simulink model "ch7example10"  (Simulink 5.0)
settings: Solver=FixedStepDiscrete  StartTime=0.0  StopTime=50  FixedStep=1e-4  RelTol=1e-3
undefined symbols (not defined in the file): rcosine
libraries: dspsigops x4, commsink2 x2, dspswit3 x1, dsparch4 x1, commcontsrc2 x1, simulink x1, commrandsrc2 x1, commutil2 x1
settings Model: LastModifiedBy=shaoyubin

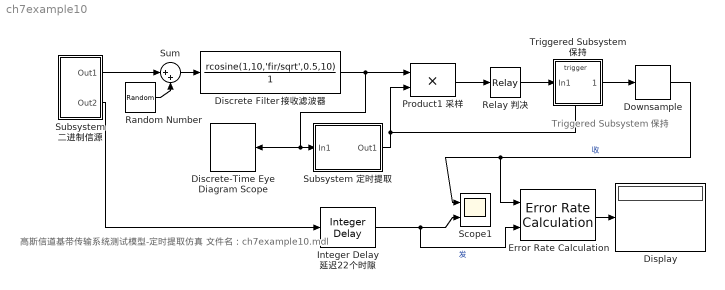
== system ch7example10 ==
  note: 高斯信道基带传输系统测试模型-定时提取仿真
      | 文件名：ch7example10.mdl
  note: Triggered
      | Subsystem
      | 保持
  Discrete Filter 接收滤波器 : DiscreteFilter  Numerator=rcosine(1,10,'fir/sqrt',0.5,10)  Denominator=1  SampleTime=1/10000
  Discrete-Time Eye Diagram Scope : commsink2/Discrete-Time Eye Diagram Scope  Tag=EyeDiagram  Orientation=left  showPlotting=on  sampPerSymb=10  offsetEye=0  symbPerTrace=2  numTraces=80  numNewFrames=80  showRendering=off  LineStyles=-  LineColors=b  dupPoints=on  fading=off  render=on  AxisGrid=on  showAxes=off  yMin=-2.17080016151619  yMax=2.13569726270215  inphaseLabel=In-phase Amplitude  quadratureLabel=Quadrature Amplitude  showFigure=off  openScopeAtSimStart=on  dispDiagram=In-phase Only  FrameNumber=on  FigPos=[76 76 560 487]  figTitle=Eye Diagram  block_type_=eye  numLinesMax=8
  Display : Display
  Downsample : dspsigops/Downsample  N=10  phase=0  ic=0  smode=Allow multirate  fmode=Maintain input frame size
  Error Rate Calculation : commsink2/Error Rate Calculation  N=0  st_delay=1  cp_mode=Entire frame  subframe=[]  PMode=Port  WsName=ErrorVec  RsMode2=off  stop=off  numErr=100  maxBits=1e6
  Integer Delay 延迟22个时隙 : dspsigops/Integer Delay  delay=22  ic=0  reset_popup=None
  Product1 采样 : Product  SaturateOnIntegerOverflow=on
  Random Number : RandomNumber  Variance=0.01  SampleTime=0
  Relay 判决 : Relay  OnSwitchValue=0  OffSwitchValue=0
  Scope1 : Scope  NumInputPorts=2
      settings: TimeRange=0.04  YMin=-2~-2  YMax=2~2
  Subsystem 定时提取 : Subsystem
  Subsystem 二进制信源 : Subsystem
  Sum : Sum  Inputs=|++  SaturateOnIntegerOverflow=on
  Triggered Subsystem 保持 : Subsystem  TreatAsAtomicUnit=on
  wires:
  Product1 采样/1 -> Relay 判决/1
  Triggered Subsystem 保持/1(Out1) -> Downsample/1
  Relay 判决/1 -> Triggered Subsystem 保持/1(In1)
  Integer Delay 延迟22个时隙/1 -> Scope1/2, Error Rate Calculation/2  "发"
  Subsystem 二进制信源/2(Out2) -> Integer Delay 延迟22个时隙/1
  Random Number/1 -> Sum/2
  Sum/1 -> Discrete Filter 接收滤波器/1
  Subsystem 二进制信源/1(Out1) -> Sum/1
  Discrete Filter 接收滤波器/1 -> Product1 采样/1, Subsystem 定时提取/1(In1), Discrete-Time Eye Diagram Scope/1
  Subsystem 定时提取/1(Out1) -> Product1 采样/2, Triggered Subsystem 保持/Trigger
  Downsample/1 -> Scope1/1, Error Rate Calculation/1  "收"
  Error Rate Calculation/1 -> Display/1

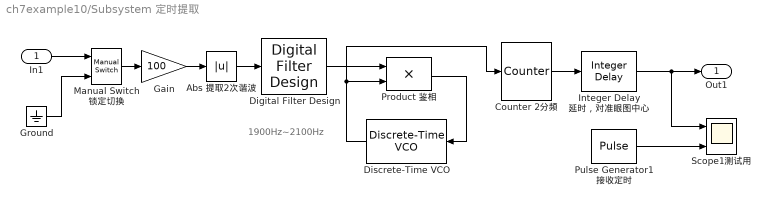
== system ch7example10/Subsystem 定时提取 ==
  note: 1900Hz~2100Hz
  In1 : Inport
  Abs 提取2次谐波 : Abs  SaturateOnIntegerOverflow=on
  Counter 2分频 : dspswit3/Counter  Direction=Up  CountEvent=Rising edge  CounterSize=User defined  MaxCount=1  InitialCount=0  Output=Count  HitValue=0  ResetInput=off  SamplesPerFrame=1  Ts=1  CntDtype=Double  HitDtype=Logical
  Digital Filter Design : dsparch4/Digital Filter Design
  Discrete-Time VCO : commcontsrc2/Discrete-Time VCO  Orientation=left  Ac=1  Fc=1998  Kc=8  Ph=0  ts=1/10000
  Gain : Gain  Gain=100  SaturateOnIntegerOverflow=on
  Ground : Ground
  Integer Delay 延时，对准眼图中心 : dspsigops/Integer Delay  delay=4  ic=0  reset_popup=None
  Manual Switch 锁定切换 : simulink/Signal Routing/Manual Switch  sw=1  action=0
  Product 鉴相 : Product  SaturateOnIntegerOverflow=on
  Pulse Generator1 接收定时 : DiscretePulseGenerator  Period=10  SampleTime=1/10000
  Scope1测试用 : Scope  NumInputPorts=2
      settings: TimeRange=0.012  YMin=-1~-1  YMax=2~2
  Out1 : Outport
  wires:
  Abs 提取2次谐波/1 -> Digital Filter Design/1
  Discrete-Time VCO/1 -> Product 鉴相/2, Counter 2分频/1
  Product 鉴相/1 -> Discrete-Time VCO/1
  Digital Filter Design/1 -> Product 鉴相/1
  Gain/1 -> Abs 提取2次谐波/1
  Manual Switch 锁定切换/1 -> Gain/1
  In1/1 -> Manual Switch 锁定切换/1
  Ground/1 -> Manual Switch 锁定切换/2
  Counter 2分频/1 -> Integer Delay 延时，对准眼图中心/1
  Integer Delay 延时，对准眼图中心/1 -> Out1/1, Scope1测试用/1
  Pulse Generator1 接收定时/1 -> Scope1测试用/2

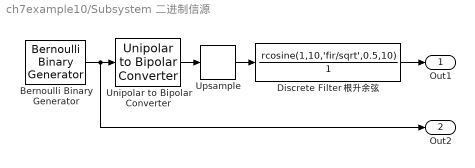
== system ch7example10/Subsystem 二进制信源 ==
  Bernoulli Binary Generator : commrandsrc2/Bernoulli Binary Generator  P=0.5  seed=61  Ts=1e-3  frameBased=off  sampPerFrame=1  orient=off
  Discrete Filter 根升余弦 : DiscreteFilter  Numerator=rcosine(1,10,'fir/sqrt',0.5,10)  Denominator=1  SampleTime=1/10000
  Unipolar to Bipolar Converter : commutil2/Unipolar to Bipolar Converter  M=2  polarity=Positive
  Upsample : dspsigops/Upsample  N=10  phase=0  ic=0  mode=Maintain input frame size
  Out1 : Outport
  Out2 : Outport  Port=2
  wires:
  Bernoulli Binary Generator/1 -> Unipolar to Bipolar Converter/1, Out2/1
  Unipolar to Bipolar Converter/1 -> Upsample/1
  Upsample/1 -> Discrete Filter 根升余弦/1
  Discrete Filter 根升余弦/1 -> Out1/1

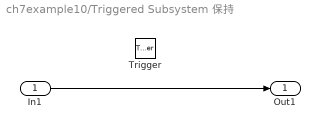
== system ch7example10/Triggered Subsystem 保持 ==
  In1 : Inport
  Trigger : TriggerPort
  Out1 : Outport
  wires:
  In1/1 -> Out1/1
